simulink model "mash111ref"  (R2024a)
settings: Solver=FixedStepDiscrete  StartTime=1  StopTime=sim_time  FixedStep=1  RelTol=1e-3  EnableMultiTasking=on
values from neighbouring files (symbols this model uses):
  M = 2^Nb    (= 1024)    [TOP.m]    (also in TOP2.m = 256; main.m; sigma_delta_sample_based.m = 512)
undefined symbols (not defined in the file or in its folder): ic1, input
settings Model: Creator=Peter Kennedy  LastModifiedBy=Peter Kennedy
settings DataIOCC: LimitDataPoints=on  SaveFormat=Array  SignalLoggingSaveFormat=ModelDataLogs  ReturnWorkspaceOutputs=off  SignalLoggingName=sigsOut
settings DebuggingCC: SaveWithParameterizedLinksMsg=none  UnderspecifiedInitializationDetection=Classic  MergeDetectMultiDrivingBlocksExec=none  SignalResolutionControl=TryResolveAllWithWarning  MultiTaskDSMMsg=warning  MultiTaskCondExecSysMsg=none  UnconnectedInputMsg=warning  UnconnectedOutputMsg=warning  UnconnectedLineMsg=warning
settings HardwareCC: ProdBitPerPointer=32  ProdBitPerSizeT=32  ProdBitPerPtrDiffT=32  ProdLargestAtomicFloat=None  ProdIntDivRoundTo=Undefined  ProdEndianess=Unspecified  ProdWordSize=32  ProdHWDeviceType=32-bit Generic  TargetUnknown=on
settings ModelReferenceCC: PropagateSignalLabelsOutOfModel=off
settings GRTTargetCC: CombineOutputUpdateFcns=off  GRTInterface=on
settings ConfigComp: CovMetricSettings=dw  CovSaveCumulativeToWorkspaceVar=on  CovSaveSingleToWorkspaceVar=on

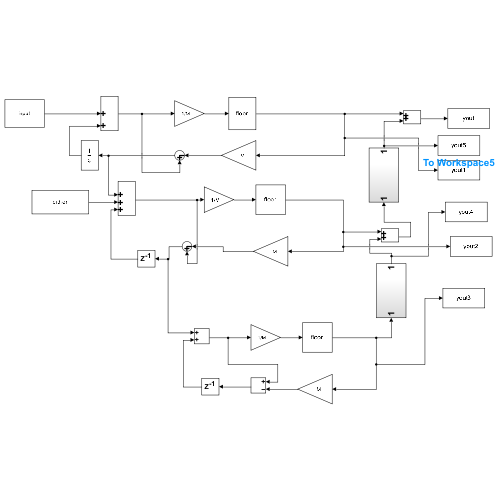
[thumbnail: Simulink's stored preview of the top-level diagram]
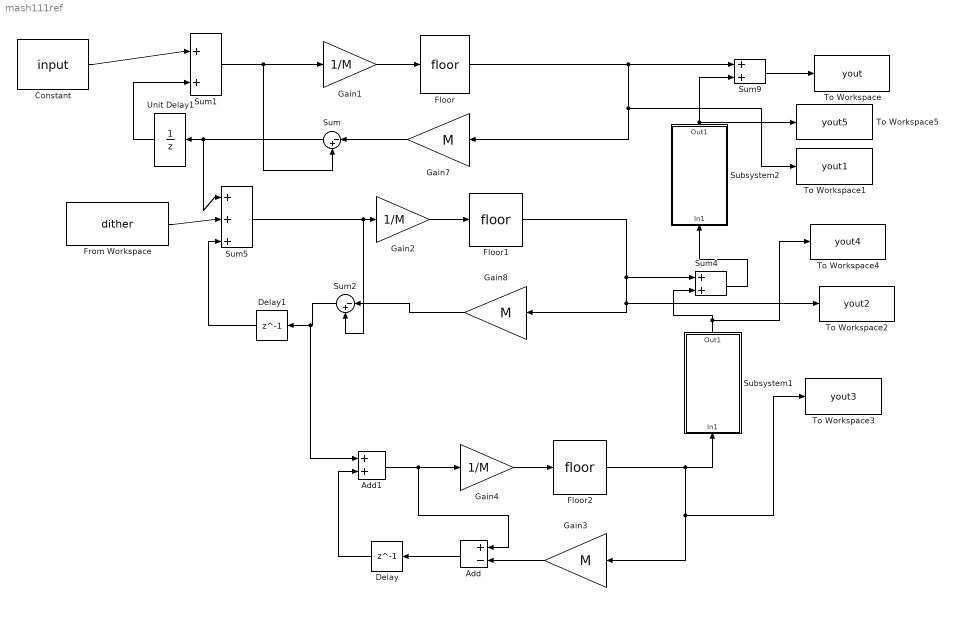
== system mash111ref ==
  Add : Sum  Inputs=+-
  Add1 : Sum
  Constant : Constant  Value=input
  Delay : Delay  DelayLength=1  InitialCondition=0
  Delay1 : Delay  DelayLength=1  InitialCondition=0
  Floor : Rounding
  Floor1 : Rounding
  Floor2 : Rounding
  From Workspace : FromWorkspace  VariableName=dither  ZeroCross=off
  Gain1 : Gain  Gain=1/M  SaturateOnIntegerOverflow=on  OutDataTypeStr=Inherit: Same as input  ParamDataTypeStr=Inherit: Same as input
  Gain2 : Gain  Gain=1/M  SaturateOnIntegerOverflow=on  OutDataTypeStr=Inherit: Same as input  ParamDataTypeStr=Inherit: Same as input
  Gain3 : Gain  Gain=M  SaturateOnIntegerOverflow=on  OutDataTypeStr=Inherit: Same as input  ParamDataTypeStr=Inherit: Same as input
  Gain4 : Gain  Gain=1/M  SaturateOnIntegerOverflow=on  OutDataTypeStr=Inherit: Same as input  ParamDataTypeStr=Inherit: Same as input
  Gain7 : Gain  Gain=M  SaturateOnIntegerOverflow=on  OutDataTypeStr=Inherit: Same as input  ParamDataTypeStr=Inherit: Same as input
  Gain8 : Gain  Gain=M  SaturateOnIntegerOverflow=on  OutDataTypeStr=Inherit: Same as input  ParamDataTypeStr=Inherit: Same as input
  Subsystem1 : Subsystem
  Subsystem2 : Subsystem
  Sum : Sum  Inputs=|-+  SaturateOnIntegerOverflow=on
  Sum1 : Sum  Inputs=|++  SaturateOnIntegerOverflow=on
  Sum2 : Sum  Inputs=|-+  SaturateOnIntegerOverflow=on
  Sum4 : Sum  SaturateOnIntegerOverflow=on
  Sum5 : Sum  Inputs=|+++  SaturateOnIntegerOverflow=on
  Sum9 : Sum  SaturateOnIntegerOverflow=on
  To Workspace : ToWorkspace  VariableName=yout  SampleTime=-1
  To Workspace1 : ToWorkspace  VariableName=yout1  SampleTime=-1
  To Workspace2 : ToWorkspace  VariableName=yout2  SampleTime=-1
  To Workspace3 : ToWorkspace  VariableName=yout3  SampleTime=-1
  To Workspace4 : ToWorkspace  VariableName=yout4  SampleTime=-1
  To Workspace5 : ToWorkspace  VariableName=yout5  SampleTime=-1
  Unit Delay1 : UnitDelay  InitialCondition=ic1
  wires:
  Gain1/1 -> Floor/1
  Sum1/1 -> Gain1/1, Sum/2
  Floor/1 -> To Workspace1/1, Gain7/1, Sum9/1
  Gain2/1 -> Floor1/1
  Sum5/1 -> Sum2/2, Gain2/1
  Subsystem2/1(Out1) -> Sum9/2, To Workspace5/1
  Sum9/1 -> To Workspace/1
  Constant/1 -> Sum1/1
  Sum/1 -> Sum5/1, Unit Delay1/1
  Gain7/1 -> Sum/1
  Gain8/1 -> Sum2/1
  Floor1/1 -> Sum4/1, To Workspace2/1, Gain8/1
  Gain4/1 -> Floor2/1
  Floor2/1 -> Subsystem1/1(In1), To Workspace3/1, Gain3/1
  Gain3/1 -> Add/2
  Add/1 -> Delay/1
  Delay/1 -> Add1/2
  Add1/1 -> Add/1, Gain4/1
  Sum2/1 -> Add1/1, Delay1/1
  Delay1/1 -> Sum5/3
  Subsystem1/1(Out1) -> To Workspace4/1, Sum4/2
  Sum4/1 -> Subsystem2/1(In1)
  Unit Delay1/1 -> Sum1/2
  From Workspace/1 -> Sum5/2

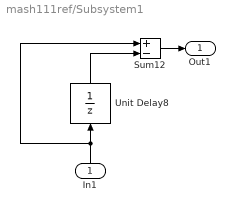
== system mash111ref/Subsystem1 ==
  In1 : Inport
  Sum12 : Sum  Inputs=+-  SaturateOnIntegerOverflow=on
  Unit Delay8 : UnitDelay
  Out1 : Outport
  wires:
  Unit Delay8/1 -> Sum12/2
  In1/1 -> Unit Delay8/1, Sum12/1
  Sum12/1 -> Out1/1

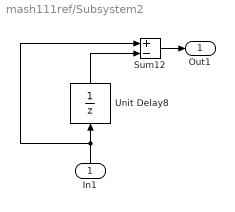
== system mash111ref/Subsystem2 ==
  In1 : Inport
  Sum12 : Sum  Inputs=+-  SaturateOnIntegerOverflow=on
  Unit Delay8 : UnitDelay
  Out1 : Outport
  wires:
  Unit Delay8/1 -> Sum12/2
  In1/1 -> Unit Delay8/1, Sum12/1
  Sum12/1 -> Out1/1
